simulink model "F16ASYM_Controlled_ACC"  (R2012b)
settings: Solver=ode3  SolverMode=SingleTasking  StartTime=0.0  StopTime=inf  FixedStep=T_sim  RelTol=1e-3
InitFcn:
  | load('NN_c_weights_Last_stable.mat')
values from neighbouring files (symbols this model uses):
  a1 = fitresult.p1    [Stall_protection.m]
  alpha_map_eval = ones(size(M_eval))*NaN    [Auto_trim_aid.m]    (also in Autotrim_maps.mat = [nan nan 0.277598136245 0.119432432992 0.0579479097061 0.027)
  beta_map_eval = ones(size(M_eval))*NaN    [Auto_trim_aid.m]    (also in Autotrim_maps.mat = [nan nan -0.00151549403324 0.00117807579006 -0.0052086799721)
  C_L_0 = fitresult.p2    [Stall_protection.m]
  G_eval = NaN*ones(size(M_sq,2),size(H_sq,2))    [Stall_protection.m]
  H_sq = unique(sort(H_sq))    [Stall_protection.m]
  H_sq_autotrim = min( F_envelope.H_1g):2000:max(F_envelope.H_1g)    [Auto_trim_aid.m]    (also in Autotrim_maps.mat = [0 2000 4000 6000 8000 10000 12000 14000 16000 18000])
  K_b_ACC = params(3)    [Cost_function.m]
  K_b_q = params(4)    [Cost_function.m]
  learning = 20    [Scheduling_desing.m]
  M_sq = unique(sort(M_sq))    [Stall_protection.m]
  M_sq_autotrim = 0:0.1:max(F_envelope.M_1g)    [Auto_trim_aid.m]    (also in Autotrim_maps.mat = [0 0.1 0.2 0.3 0.4 0.5 0.6 0.7 0.8 0.9 1 1.1 ... (21 element)
  Model_used_flag = 1    [Scheduling_desing.m]
  reg_param = 1    [Scheduling_desing.m]
  T_sim = 0.04    [Run_me.m]    (also in Scheduling_desing.m = 0.02)
  tau_ACC = params(1)    [Cost_function.m]
  tau_q = params(2)    [Cost_function.m]
  V_Comp_A_w_z_last = [-0.043311742939 0.0085685727899 -0.0213735657625 0.0330213821126 -0.0306555996667 -0.00573122365227 -0.0106441480787 0.0329440631876 0.0177121952361 -0.0290685435098 -0.0181457235686 -0.0361990502411 ... (1250 elements, 50x25)]    [NN_c_weights_Last_stable.mat]
  V_Comp_last = [-0.0421958473648 0.0184516098779 -0.0436695953504 -0.041154016657 0.00216882652165 -0.0388561228631 0.0327521861474 0.0326079628857 0.0227071838361 -0.0338588476214 0.0161615063846 0.00186003522421 ... (1250 elements, 50x25)]    [NN_c_weights_Last_stable.mat]
  velocity = M_eval(I,J)*a    [Auto_trim_aid.m]    (also in Scheduling_desing.m = M_eval_sche(I,J)*a)
  W_Comp_A_w_z_last = [-0.00689921461652 0.00234704735165 -0.000126421245896 0.00121944724496 6.17702028018e-05 -0.000422762754226 -0.000228913732743 -1.1618795843e-05 7.94007436465e-05 0.000588815786054 2.98617078429e-05 -0.00020420127191 ... (153 elements, 3x51)]    [NN_c_weights_Last_stable.mat]
  W_Comp_last = [-0.00864477030284 0.000183920433695 -0.000300268209456 0.00178165628538 -0.000144806488148 -0.000715209966 -0.000733452792184 5.9552378004e-05 0.000293789747621 0.00184648331608 -0.000150090451416 -0.000741280397229 ... (153 elements, 3x51)]    [NN_c_weights_Last_stable.mat]
undefined symbols (not defined in the file or in its folder): B, DiscIntNeverNeededParam, fi_flag_Simulink, k_B, m_B, sigbuilder_block, Stall_curve, Theta_1_roll_last, Theta_2_roll_last, Theta_3_roll_last, trim_control, trim_state, trim_throttle, V_long_lastA_w_z, V_long_lastAoA, V_roll_last, V_roll_lastMOD, V_yaw_last, W_long_lastA_w_z, W_long_lastAoA, W_roll_last, W_roll_lastMOD, W_yaw_last
libraries: Adaptive_FaultTolerantControl x43, F16_Actuator_Library x14, dspsigops x13, simulink x8, dsparch4 x6, simulink_extras x5, aerolibatmos2 x5, aerolibtransform2 x5, dspmtrx3 x3, qcatlib x2, dspvision x2, dspsnks4 x2
(part 9 of 10)

== system F16ASYM_Controlled_ACC/Primary Controller/P controller + adaptive Crossed NN/Longitudinal Controller: AoA or A_w_z/Longitudinal controller in A_w_z/Accel rate --> AoA rate! ==
  All_meas : Inport
  1/a_1 : Gain  Gain=1/a1
  Bus Selector : BusSelector  OutputSignals=signal2.q (Pa)
  Divide : Product  Inputs=**
  Divide2 : Product  Inputs=*/
  S : Constant  Value=27.87
  mass : Constant  Value=9295.44
  A_w  to AoA rates factor : Outport
  wires:
  1/a_1/1 -> A_w  to AoA rates factor/1
  All_meas/1 -> Bus Selector/1
  Divide2/1 -> 1/a_1/1
  Divide/1 -> Divide2/2
  mass/1 -> Divide2/1
  Bus Selector/1 -> Divide/2  "<q (Pa)>"
  S/1 -> Divide/1

== system F16ASYM_Controlled_ACC/Primary Controller/P controller + adaptive Crossed NN + AWU+Lim /Longitudinal Controller: AoA or A_w_z/Longitudinal controller in A_w_z/Accel rate --> AoA rate! ==
  All_meas : Inport
  1/a_1 : Gain  Gain=1/a1
  Bus Selector : BusSelector  OutputSignals=signal2.q (Pa)
  Divide : Product  Inputs=**
  Divide2 : Product  Inputs=*/
  S : Constant  Value=27.87
  mass : Constant  Value=9295.44
  A_w  to AoA rates factor : Outport
  wires:
  S/1 -> Divide/1
  Bus Selector/1 -> Divide/2  "<q (Pa)>"
  mass/1 -> Divide2/1
  Divide/1 -> Divide2/2
  Divide2/1 -> 1/a_1/1
  All_meas/1 -> Bus Selector/1
  1/a_1/1 -> A_w  to AoA rates factor/1

== matlab function F16ASYM_Controlled_ACC/P controller + adaptive Crossed NN + AWU+Lim    in ACC /Complete crossed On-line (adaptive) multi-layer NN: A_w_z/Cross NN A_w_z ==
  data: X_bar input size=[25,1]; v_ad_comp output; e input; Factor_F input; K_roll input; Ks_long input; Ks_yaw input; B input; Learnign_rate input size=1; Reg_param input size=1; AWU input; W input size=[3,51]; V input size=[50,25]; v_ad output; Z_norm_unit output; T_sim parameter; W_update output; V_update output
function [v_ad_comp,v_ad,Z_norm_unit,W_update,V_update]  = Cross_NN(X_bar,e,Factor_F, K_roll,Ks_long,Ks_yaw,B,Learnign_rate,Reg_param,AWU,W,V,T_sim)

%% Compute prelimiary parametes
% Compute P with regular Lyapunov equation solution
P_roll=1/K_roll;
P_long =  [   1/Ks_long(1) , Factor_F/(Ks_long(1)^2+Ks_long(1)*Ks_long(2));
     1/(Ks_long(1)^2+Ks_long(1)*Ks_long(2)) ,(Ks_long(1)^2+Ks_long(1)*Ks_long(2)+Factor_F^2)/(Ks_long(2)^2*Ks_long(1)+Ks_long(2)*Ks_long(1)^2) ];
P_yaw = [   1/Ks_yaw(1) , 1/(Ks_yaw(1)^2+Ks_yaw(1)*Ks_yaw(2));
     1/(Ks_yaw(1)^2+Ks_yaw(1)*Ks_yaw(2)) ,(Ks_yaw(1)^2+Ks_yaw(1)*Ks_yaw(2)+1)/(Ks_yaw(2)^2*Ks_yaw(1)+Ks_yaw(2)*Ks_yaw(1)^2) ];
 
P = blkdiag(P_roll,P_long,P_yaw);

% % % % Compute P with on-line Lyapunov equation solution
% % % CROSS = 0;
% % % A = [ -K_roll,0,CROSS,0,0;0,-Ks_long(1),1,0,0;
% % %     0,0,-Ks_long(2),0,0;0,0,0,-Ks_yaw(1),Factor_F;0,0,0,0,-Ks_yaw(2)];
% % % 
% % % coder.extrinsic('lyap')
% % % P = A;
% % % P = lyap(A,2*diag(ones(5,1)));



K_awu = 1.2;
zeta= e'*P*B;


% Introduce Anti-windup
zeta = zeta - K_awu*AWU'.*T_sim; 

% Convergence limitation
if norm(zeta)>2/(T_sim*Learnign_rate*Reg_param)
    zeta = (zeta./norm(zeta)).*(1.8/(T_sim*Learnign_rate*Reg_param));
end

%% Feedforward
z = V*X_bar;
s=sigmoid(V*X_bar);

sigma = [1 ; s ];
% v_ad = W*sigma;

sigma_grad = (sigma.*(ones(size(sigma))-sigma));

%% Compute the gradients or adaptation laws
Gamma_w= Learnign_rate; % W learnign rate
Gamma_v= Learnign_rate; %V learning rate
lambda = Reg_param;

V_dot=zeros(size(V));
W_dot=zeros(size(W));

W_dot= -Gamma_w*(  (sigma - sigma_grad.*[1;z] )*zeta  )';
W_dot(:,2:end)= W_dot(:,2:end) - Gamma_w*lambda*norm(zeta)*(W(:,2:end));

M = W'*zeta'.*sigma_grad ;
V_dot= -Gamma_v*( M(2:end)*X_bar'  );
V_dot(:,2:end)= V_dot(:,2:end) - Gamma_v*lambda*norm(zeta).*V(:,2:end);

% % % Other way: Based on notes of Andrew NG
% % 
% % delta2=W'*zeta'.*sigma_grad;
% % 
% % V_dot = - Gamma_v*( delta2(2:end)*X_bar');
% % V_dot(:,2:end)= V_dot(:,2:end) - Gamma_v*lambda*norm(zeta).*V(:,2:end);
% % 
% % W_dot = - Gamma_w*( sigma*zeta)';
% % W_dot(:,2:end)= W_dot(:,2:end) - Gamma_w*lambda*norm(zeta)*(W(:,2:end));



%% Adaptation
W_update = W + T_sim*W_dot;
V_update = V + T_sim*V_dot;
% 
%% Re-compute v_ad

s=sigmoid(V_update*X_bar);

sigma = [1 ; s(:,1) ];
v_ad = W_update*sigma;

%% Compute v_ad_comp
Z = [ V,zeros(size(V,1),size(W,2));
    zeros(size(W,1),size(V,2)),W];
    
Z_norm = norm(Z,'fro');
Z_max = 2*min(size(W,1),size(W,2) )*min( size(V,1),size(V,2) );
Z_norm_unit = Z_norm;

K_r0= 0;
K_r1= 0;
v_r0 = -K_r0*zeta';
v_r1 = -K_r1*(Z_norm+Z_max)*zeta';

v_ad_comp = v_ad + v_r1 +v_r0;

% % % Normalization of matrices
% % if Z_norm>Z_max
% %     V = (V.*Z_max)./Z_norm;
% %     W = (W.*Z_max)./Z_norm;
% % end
end

== matlab function F16ASYM_Controlled_ACC/Primary Controller/P  + Crossed NN + AWU+Lim + hand-over/P controller + adaptive Crossed NN + AWU+Lim   in AoA/Physical limitation/max deflections estimator ==
  data: v_comm input; max_defl output; B parameter
function max_defl = Max_defl(v_comm,B)
sup_limit = [24,24,21,21,29,25,25];
inf_limit = [-24,-24,-21,-21,-29,0,0];

def=B;
for i=1:3
    def(i,:) = B(i,:).*sign(v_comm(i));
end
def_avg = mean(def,1);

max_defl = zeros(7,1);
for i=1:7
    if def_avg(1,i)>0
        max_defl(i) = sup_limit(i);
    else
        max_defl(i) = inf_limit(i);
    end
end

== matlab function F16ASYM_Controlled_ACC/Primary Controller/P  + Crossed NN + AWU+Lim + hand-over/P controller + adaptive Crossed NN + AWU+Lim    in ACC /Physical limitation/max deflections estimator ==
  data: v_comm input; max_defl output; B parameter
function max_defl = Max_defl(v_comm,B)
sup_limit = [24,24,21,21,29,25,25];
inf_limit = [-24,-24,-21,-21,-29,0,0];

def=B;
for i=1:3
    def(i,:) = B(i,:).*sign(v_comm(i));
end
def_avg = mean(def,1);

max_defl = zeros(7,1);
for i=1:7
    if def_avg(1,i)>0
        max_defl(i) = sup_limit(i);
    else
        max_defl(i) = inf_limit(i);
    end
end

== matlab function F16ASYM_Controlled_ACC/P controller + adaptive Crossed NN + AWU+Lim    in ACC /Sigmoid /MATLAB Function ==
  data: u input; y output; a input
function y = sigmoid_a(u,a)

y = 2.0 ./ (1.0 + exp(-a*u(1:3)))-1;

== system F16ASYM_Controlled_ACC/Primary Controller/P controller + adaptive Crossed NN + AWU+Lim /Longitudinal Controller: AoA or A_w_z/Longitudinal controller in A_w_z/Stall protection ==
  alpha_dot des : Inport
  All meas : Inport  Port=2
  Bus Selector : BusSelector  OutputSignals=signal1.AoA meas (rad)
  MATLAB Function : MATLAB Function  TreatAsAtomicUnit=on
  AoA des : Outport
  wires:
  alpha_dot des/1 -> MATLAB Function/1(alpha_dot)
  MATLAB Function/1(alpha_dot_out) -> AoA des/1
  All meas/1 -> Bus Selector/1
  Bus Selector/1 -> MATLAB Function/2(alpha)  "<AoA meas (rad)>"

== system F16ASYM_Controlled_ACC/Primary Controller/P controller + adaptive Isolated NN/Longitudinal Controller: AoA or A_w_z/Longitudinal controller in A_w_z/Accel rate --> AoA rate! ==
  All_meas : Inport
  1/a_1 : Gain  Gain=1/a1
  Bus Selector : BusSelector  OutputSignals=signal2.q (Pa)
  Divide : Product  Inputs=**
  Divide2 : Product  Inputs=*/
  S : Constant  Value=27.87
  mass : Constant  Value=9295.44
  A_w  to AoA rates factor : Outport
  wires:
  S/1 -> Divide/1
  Bus Selector/1 -> Divide/2  "<q (Pa)>"
  mass/1 -> Divide2/1
  Divide/1 -> Divide2/2
  Divide2/1 -> 1/a_1/1
  All_meas/1 -> Bus Selector/1
  1/a_1/1 -> A_w  to AoA rates factor/1

== system F16ASYM_Controlled_ACC/Primary Controller/P controller + adaptive Isolated NN/On-line (adaptive) multi-layer NNs/Long Chanel/Long HL NN A_w_z ==
  note: Be careful with dimensions of inputs!!!
      | NORMALIZATION!!!
  v_ad^ prev : Inport
  Long_chanel vars : Inport  Port=2
  All_meas : Inport  Port=3
  Long_learning rate : Inport  Port=4
  Long reg param : Inport  Port=5
  Bus Selector1 : BusSelector  OutputSignals=A_chanel vars.A_err,q_chanel_vars.q_err,A_chanel vars.A_sf,A_chanel vars.A_sf_dot,q_chanel_vars.q_sf_dot,A_chanel vars.K_b_A,q_chanel_vars.K_b_q,A_chanel vars.FactorF
  Bus Selector2 : BusSelector  OutputSignals=signal1.Alt meas (m),signal2.Mach
  Constant : Constant
  Constant1 : Constant  Value=[0;1]
  Divide : Product  Inputs=**
  Long NN : MATLAB Function  TreatAsAtomicUnit=on
  Memory2 : Memory  X0=V_long_lastA_w_z
  Memory3 : Memory  X0=W_long_lastA_w_z
  Mux : Mux  Inputs=10
  Mux1 : Mux  Inputs=2
  Mux2 : Mux  Inputs=2
  Scope : Scope
      settings: YMin=0  YMax=0.003  SaveName=ScopeData13
  Terminator : Terminator
  Terminator1 : Terminator
  To Workspace : ToWorkspace  VariableName=V_long_lastA_w_z  SampleTime=-1
      settings: MaxDataPoints=1
  To Workspace1 : ToWorkspace  VariableName=W_long_lastA_w_z  SampleTime=-1
      settings: MaxDataPoints=1
  dim-less : Gain  Gain=T_sim
  dim-less1 : Gain  Gain=T_sim^2
  scaling : Gain  Gain=1/15000
  scaling1 : Gain  Gain=1/(9*9.81)
  scaling2 : Gain  Gain=1/(9*9.81)
  scaling3 : Gain  Gain=1/(9*9.81)
  v_ad_comp : Outport
  wires:
  Long NN/2(v_ad) -> Terminator/1
  Long NN/5(V_update) -> To Workspace/1, Memory2/1
  v_ad^ prev/1 -> Mux/10
  [Ks] -> Long NN/4(Ks)
  Constant1/1 -> Long NN/5(B)
  Memory3/1 -> Long NN/8(W)
  Memory2/1 -> Long NN/9(V)
  Long NN/4(W_update) -> To Workspace1/1, Memory3/1
  Long NN/1(v_ad_comp) -> v_ad_comp/1
  Mux/1 -> Scope/1, Long NN/1(X_bar)
  Long_chanel vars/1 -> Bus Selector1/1
  Long_learning rate/1 -> Long NN/6(Long_learnign_rate)
  Long reg param/1 -> Long NN/7(Long_reg_param)
  Constant/1 -> Mux/1
  All_meas/1 -> Bus Selector2/1
  Bus Selector2/1 -> scaling/1  "<Alt meas (m)>"
  Divide/1 -> Mux/4
  scaling/1 -> Mux/2
  Bus Selector2/2 -> Mux/3, Divide/2, Divide/1  "<Mach>"
  Bus Selector1/1 -> Mux1/1, scaling2/1  "<A_err>"
  Bus Selector1/2 -> Mux1/2, Mux/6  "<q_err>"
  Bus Selector1/3 -> scaling1/1  "<A_sf>"
  Bus Selector1/4 -> dim-less/1  "<A_sf_dot>"
  Bus Selector1/5 -> dim-less1/1  "<q_sf_dot>"
  Mux1/1 -> Long NN/2(e)  "e"
  Bus Selector1/7 -> Mux2/2  "<K_b_q>"
  Bus Selector1/6 -> Mux2/1  "<K_b_A>"
  Mux2/1 -> [Ks]
  Bus Selector1/8 -> Long NN/3(F)  "<FactorF>"
  scaling2/1 -> Mux/5
  scaling1/1 -> Mux/7
  scaling3/1 -> Mux/8
  Long NN/3(Z_norm_unit) -> Terminator1/1
  dim-less/1 -> scaling3/1
  dim-less1/1 -> Mux/9

== system F16ASYM_Controlled_ACC/Primary Controller/P controller + adaptive Isolated NN/On-line (adaptive) multi-layer NNs/Long Chanel/Long HL NN AoA ==
  note: Be careful with dimensions of inputs!!!
      | NORMALIZATION!!!
  v_ad^ prev : Inport
  Long_chanel vars : Inport  Port=2
  All_meas : Inport  Port=3
  Long_learning rate : Inport  Port=4
  Long reg param : Inport  Port=5
  Bus Selector1 : BusSelector  OutputSignals=alpha_chanel vars.alpha_err,q_chanel_vars.q_err,alpha_chanel vars.alpha_sf,alpha_chanel vars.alpha_sf_dot,q_chanel_vars.q_sf_dot,alpha_chanel vars.K_b_alpha,q_chanel_vars.K_b_q
  Bus Selector2 : BusSelector  OutputSignals=signal1.Alt meas (m),signal2.Mach
  Constant : Constant
  Constant1 : Constant  Value=[0;1]
  Display : Display
  Divide : Product  Inputs=**
  Gain : Gain  Gain=1/15000
  Long NN : MATLAB Function  TreatAsAtomicUnit=on
  Memory2 : Memory  X0=V_long_lastAoA
  Memory3 : Memory  X0=W_long_lastAoA
  Mux : Mux  Inputs=10
  Mux1 : Mux  Inputs=2
  Mux2 : Mux  Inputs=2
  Scope : Scope
      settings: YMin=-0.7  YMax=1  SaveName=ScopeData18
  Terminator : Terminator
  Terminator1 : Terminator
  To Workspace : ToWorkspace  VariableName=V_long_lastAoA  SampleTime=-1
      settings: MaxDataPoints=1
  To Workspace1 : ToWorkspace  VariableName=W_long_lastAoA  SampleTime=-1
      settings: MaxDataPoints=1
  dem-less : Gain  Gain=T_sim
  dem-less1 : Gain  Gain=T_sim^2
  v_ad_comp : Outport
  wires:
  Long NN/2(v_ad) -> Terminator/1
  Long NN/5(V_update) -> To Workspace/1, Memory2/1
  v_ad^ prev/1 -> Mux/10
  [Ks] -> Long NN/3(Ks)
  Constant1/1 -> Long NN/4(B)
  Memory3/1 -> Long NN/7(W)
  Memory2/1 -> Long NN/8(V)
  Long NN/4(W_update) -> To Workspace1/1, Memory3/1
  Long NN/1(v_ad_comp) -> v_ad_comp/1
  Long_chanel vars/1 -> Bus Selector1/1
  Long_learning rate/1 -> Long NN/5(Long_learnign_rate)
  Long reg param/1 -> Long NN/6(Long_reg_param)
  Constant/1 -> Mux/1
  All_meas/1 -> Bus Selector2/1
  Bus Selector2/1 -> Gain/1  "<Alt meas (m)>"
  Divide/1 -> Mux/4
  Gain/1 -> Mux/2
  Bus Selector2/2 -> Mux/3, Divide/2, Divide/1  "<Mach>"
  Bus Selector1/1 -> Mux1/1, Mux/5  "<alpha_err>"
  Bus Selector1/2 -> Mux1/2, Mux/6  "<q_err>"
  Bus Selector1/3 -> Mux/7  "<alpha_sf>"
  Bus Selector1/4 -> dem-less/1  "<alpha_sf_dot>"
  Bus Selector1/5 -> dem-less1/1  "<q_sf_dot>"
  Mux1/1 -> Long NN/2(e)  "e"
  Bus Selector1/7 -> Mux2/2  "<K_b_q>"
  Bus Selector1/6 -> Mux2/1  "<K_b_alpha>"
  Mux2/1 -> [Ks]
  Long NN/3(Z_norm_unit) -> Terminator1/1
  Mux/1 -> Scope/1, Display/1, Long NN/1(X_bar)
  dem-less/1 -> Mux/8
  dem-less1/1 -> Mux/9

== system F16ASYM_Controlled_ACC/Primary Controller/P controller + adaptive Isolated NN/On-line (adaptive) multi-layer NNs/Roll NN/Roll 1HL NN ==
  note: Be careful with dimensions of inputs!!!
      | NORMALIZATION!!!
  v_ad^ prev : Inport
  p_chanel vars : Inport  Port=2
  All_meas : Inport  Port=3
  Roll_learning rate : Inport  Port=4
  Roll reg param : Inport  Port=5
  Bus Selector1 : BusSelector  OutputSignals=p_err,p_sf,p_sf_dot,K_b_p
  Bus Selector2 : BusSelector  OutputSignals=signal1.Alt meas (m),signal2.Mach,signal1.AoA meas (rad),signal1.SS meas (rad),signal1.omega_b meas (rad/s)
  Constant : Constant
  Constant1 : Constant
  Constant2 : Constant
  Display : Display
  Divide : Product  Inputs=**
  Divide1 : Product  Inputs=**
  Divide2 : Product  Inputs=*/
  Memory2 : Memory  X0=V_roll_last
  Memory3 : Memory  X0=W_roll_last
  Mux : Mux  Inputs=12
  Roll NN : MATLAB Function  TreatAsAtomicUnit=on
  Scope : Scope
      settings: YMin=-0.5  YMax=6  SaveName=ScopeData15
  Selector : Selector  InputPortWidth=3  IndexOptions=Index vector (dialog)  Indices=3  OutputSizes=1
  Terminator : Terminator
  Terminator1 : Terminator
  To Workspace : ToWorkspace  VariableName=V_roll_last  SampleTime=-1
      settings: MaxDataPoints=1
  To Workspace1 : ToWorkspace  VariableName=W_roll_last  SampleTime=-1
      settings: MaxDataPoints=1
  dem-less : Gain  Gain=T_sim
  dim-less : Gain  Gain=1/15000
  v_ad_comp : Outport
  wires:
  Constant2/1 -> Divide2/1
  Bus Selector1/4 -> Divide2/2  "<K_b_p>"
  Divide2/1 -> [P]
  Roll NN/2(v_ad) -> Terminator/1
  Roll NN/5(V_update) -> To Workspace/1, Memory2/1
  v_ad^ prev/1 -> Mux/12
  [P] -> Roll NN/3(P)
  Constant1/1 -> Roll NN/4(B)
  Memory3/1 -> Roll NN/7(W)
  Memory2/1 -> Roll NN/8(V)
  Roll NN/4(W_update) -> To Workspace1/1, Memory3/1
  Roll NN/1(v_ad_comp) -> v_ad_comp/1
  Mux/1 -> Roll NN/1(X_bar), Scope/1, Display/1
  Bus Selector1/1 -> Mux/9, Roll NN/2(e)  "<p_err>"
  Bus Selector1/3 -> dem-less/1  "<p_sf_dot>"
  Bus Selector1/2 -> Mux/10  "<p_sf>"
  p_chanel vars/1 -> Bus Selector1/1
  Roll_learning rate/1 -> Roll NN/5(Roll_learnign_rate)
  Roll reg param/1 -> Roll NN/6(Roll_reg_param)
  Constant/1 -> Mux/1
  All_meas/1 -> Bus Selector2/1
  Bus Selector2/1 -> dim-less/1  "<Alt meas (m)>"
  Divide/1 -> Mux/4
  Bus Selector2/3 -> Divide1/2, Divide1/1, Mux/5  "<AoA meas (rad)>"
  Divide1/1 -> Mux/6
  Bus Selector2/4 -> Mux/7  "<SS meas (rad)>"
  dim-less/1 -> Mux/2
  Bus Selector2/5 -> Selector/1  "<omega_b meas (rad/s)>"
  Selector/1 -> Mux/8
  Bus Selector2/2 -> Divide/2, Divide/1, Mux/3  "<Mach>"
  Roll NN/3(Z_norm_unit) -> Terminator1/1
  dem-less/1 -> Mux/11

== system F16ASYM_Controlled_ACC/Primary Controller/P controller + adaptive Isolated NN/On-line (adaptive) multi-layer NNs/Roll NN/Roll 2HL NN ==
  note: Be careful with dimensions of inputs!!!
      | NORMALIZATION!!!
  v_ad^ prev : Inport
  p_chanel vars : Inport  Port=2
  All_meas : Inport  Port=3
  Roll_learning rate : Inport  Port=4
  Roll reg param : Inport  Port=5
  " " : ToWorkspace  VariableName=Theta_3_roll_last  SampleTime=-1
      settings: MaxDataPoints=1
  "  " : Memory  X0=Theta_3_roll_last
  "   " : Memory  X0=Theta_2_roll_last
  B : Constant
  Bus Selector1 : BusSelector  OutputSignals=p_err,p_sf,p_sf_dot,K_b_p
  Bus Selector2 : BusSelector  OutputSignals=signal1.Alt meas (m),signal2.Mach,signal1.AoA meas (rad),signal1.SS meas (rad),signal1.omega_b meas (rad/s)
  Constant : Constant
  Constant2 : Constant
  Display : Display
  Divide : Product  Inputs=**
  Divide1 : Product  Inputs=**
  Divide2 : Product  Inputs=*/
  Gain : Gain  Gain=1/15000
  Memory2 : Memory  X0=Theta_1_roll_last
  Mux : Mux  Inputs=12
  Roll Multilayer NN : MATLAB Function  TreatAsAtomicUnit=on
  Scope : Scope
      settings: YMin=-14  YMax=4  SaveName=ScopeData16
  Selector : Selector  InputPortWidth=3  IndexOptions=Index vector (dialog)  Indices=3  OutputSizes=1
  Terminator : Terminator
  Terminator1 : Terminator
  To Workspace : ToWorkspace  VariableName=Theta_1_roll_last  SampleTime=-1
      settings: MaxDataPoints=1
  To Workspace1 : ToWorkspace  VariableName=Theta_2_roll_last  SampleTime=-1
      settings: MaxDataPoints=1
  dem-less : Gain  Gain=T_sim
  v_ad_comp : Outport
  wires:
  p_chanel vars/1 -> Bus Selector1/1
  Bus Selector1/2 -> Mux/10  "<p_sf>"
  Bus Selector1/3 -> dem-less/1  "<p_sf_dot>"
  Bus Selector1/1 -> Mux/9, Roll Multilayer NN/2(e)  "<p_err>"
  Constant/1 -> Mux/1
  All_meas/1 -> Bus Selector2/1
  Bus Selector2/1 -> Gain/1  "<Alt meas (m)>"
  Divide/1 -> Mux/4
  Bus Selector2/3 -> Divide1/2, Divide1/1, Mux/5  "<AoA meas (rad)>"
  Divide1/1 -> Mux/6
  Bus Selector2/4 -> Mux/7  "<SS meas (rad)>"
  Gain/1 -> Mux/2
  Bus Selector2/5 -> Selector/1  "<omega_b meas (rad/s)>"
  Selector/1 -> Mux/8
  Roll Multilayer NN/1(v_ad_comp) -> v_ad_comp/1
  "   "/1 -> Roll Multilayer NN/8(Theta_2)
  B/1 -> Roll Multilayer NN/4(B)
  [P] -> Roll Multilayer NN/3(P)
  v_ad^ prev/1 -> Mux/12
  Roll Multilayer NN/4(Theta_1_update) -> To Workspace/1, Memory2/1
  Roll Multilayer NN/2(v_ad) -> Terminator/1
  Divide2/1 -> [P]
  Bus Selector1/4 -> Divide2/2  "<K_b_p>"
  Constant2/1 -> Divide2/1
  Bus Selector2/2 -> Divide/2, Divide/1, Mux/3  "<Mach>"
  Roll Multilayer NN/6(Theta_3_update) -> "  "/1, " "/1
  "  "/1 -> Roll Multilayer NN/9(Theta_3)
  Roll Multilayer NN/5(Theta_2_update) -> To Workspace1/1, "   "/1
  Memory2/1 -> Roll Multilayer NN/7(Theta_1)
  Roll_learning rate/1 -> Roll Multilayer NN/5(Roll_learnign_rate)
  Roll reg param/1 -> Roll Multilayer NN/6(Roll_reg_param)
  Mux/1 -> Display/1, Scope/1, Roll Multilayer NN/1(X_bar)
  Roll Multilayer NN/3(Z_norm_unit) -> Terminator1/1
  dem-less/1 -> Mux/11

== system F16ASYM_Controlled_ACC/Primary Controller/P controller + adaptive Isolated NN/On-line (adaptive) multi-layer NNs/Yaw Chanel/Yaw HL NN ==
  note: Be careful with dimensions of inputs!!!
      | NORMALIZATION!!!
  v_ad^ prev : Inport
  Yaw_chanel vars : Inport  Port=2
  All_meas : Inport  Port=3
  Yaw_learning rate : Inport  Port=4
  Yaw reg param : Inport  Port=5
  Bus Selector1 : BusSelector  OutputSignals=beta_chanel vars.beta_err,r_chanel vars.r_err,beta_chanel vars.beta_sf,beta_chanel vars.beta_sf_dot,r_chanel vars.r_sf_dot,beta_chanel vars.K_b_beta,r_chanel vars.K_b_r
  Bus Selector2 : BusSelector  OutputSignals=signal1.Alt meas (m),signal2.Mach,signal1.AoA meas (rad),signal1.Euler meas (rad)
  Constant : Constant
  Constant1 : Constant  Value=[0;1]
  Display : Display
  Divide : Product  Inputs=**
  Gain : Gain  Gain=1/15000
  Memory2 : Memory  X0=V_yaw_last
  Memory3 : Memory  X0=W_yaw_last
  Mux : Mux  Inputs=12
  Mux1 : Mux  Inputs=2
  Mux2 : Mux  Inputs=2
  Scope : Scope
      settings: YMin=-0.25  YMax=3.75  SaveName=ScopeData17
  Selector : Selector  InputPortWidth=3  IndexOptions=Index vector (dialog)  Indices=1  OutputSizes=1
  Terminator : Terminator
  Terminator1 : Terminator
  To Workspace : ToWorkspace  VariableName=V_yaw_last  SampleTime=-1
      settings: MaxDataPoints=1
  To Workspace1 : ToWorkspace  VariableName=W_yaw_last  SampleTime=-1
      settings: MaxDataPoints=1
  Yaw NN : MATLAB Function  TreatAsAtomicUnit=on
  dem-less1 : Gain  Gain=T_sim
  dem-less2 : Gain  Gain=T_sim^2
  v_ad_comp : Outport
  wires:
  Mux2/1 -> [Ks]
  Bus Selector1/6 -> Mux2/1  "<K_b_beta>"
  Bus Selector1/7 -> Mux2/2  "<K_b_r>"
  Mux1/1 -> Yaw NN/2(e)  "e"
  Divide/1 -> Mux/4
  Bus Selector2/1 -> Gain/1  "<Alt meas (m)>"
  All_meas/1 -> Bus Selector2/1
  Constant/1 -> Mux/1
  Yaw reg param/1 -> Yaw NN/6(Long_reg_param)
  Yaw_learning rate/1 -> Yaw NN/5(Long_learnign_rate)
  Yaw_chanel vars/1 -> Bus Selector1/1
  Yaw NN/1(v_ad_comp) -> v_ad_comp/1
  Yaw NN/4(W_update) -> Memory3/1, To Workspace1/1
  Memory2/1 -> Yaw NN/8(V)
  Memory3/1 -> Yaw NN/7(W)
  Constant1/1 -> Yaw NN/4(B)
  [Ks] -> Yaw NN/3(Ks)
  v_ad^ prev/1 -> Mux/12
  Yaw NN/5(V_update) -> Memory2/1, To Workspace/1
  Yaw NN/2(v_ad) -> Terminator/1
  Bus Selector2/4 -> Selector/1  "<Euler meas (rad)>"
  Gain/1 -> Mux/2
  Bus Selector2/2 -> Divide/2, Divide/1, Mux/3  "<Mach>"
  Bus Selector2/3 -> Mux/5  "<AoA meas (rad)>"
  Selector/1 -> Mux/6
  Bus Selector1/5 -> dem-less2/1  "<r_sf_dot>"
  Bus Selector1/2 -> Mux1/2, Mux/8  "<r_err>"
  Bus Selector1/4 -> dem-less1/1  "<beta_sf_dot>"
  Bus Selector1/1 -> Mux1/1, Mux/7  "<beta_err>"
  Bus Selector1/3 -> Mux/9  "<beta_sf>"
  Mux/1 -> Display/1, Scope/1, Yaw NN/1(X_bar)
  Yaw NN/3(Z_norm_unit) -> Terminator1/1
  dem-less1/1 -> Mux/10
  dem-less2/1 -> Mux/11

== system F16ASYM_Controlled_ACC/Primary Controller/P controller + adaptive Isolated NN/On-line (adaptive) multi-layer NNs SIMPL/Long Chanel/Long HL NN A_w_z ==
  note: Be careful with dimensions of inputs!!!
      | NORMALIZATION!!!
  v_ad^ prev : Inport
  Long_chanel vars : Inport  Port=2
  All_meas : Inport  Port=3
  Long_learning rate : Inport  Port=4
  Long reg param : Inport  Port=5
  Bus Selector1 : BusSelector  OutputSignals=A_chanel vars.A_err,q_chanel_vars.q_err,A_chanel vars.A_sf,A_chanel vars.A_sf_dot,q_chanel_vars.q_sf_dot,A_chanel vars.K_b_A,q_chanel_vars.K_b_q,A_chanel vars.FactorF
  Bus Selector2 : BusSelector  OutputSignals=signal1.Alt meas (m),signal2.Mach
  Constant : Constant
  Constant1 : Constant  Value=[0;1]
  Divide : Product  Inputs=**
  Long NN : MATLAB Function  TreatAsAtomicUnit=on
  Memory2 : Memory  X0=V_long_lastA_w_z
  Memory3 : Memory  X0=W_long_lastA_w_z
  Mux : Mux  Inputs=10
  Mux1 : Mux  Inputs=2
  Mux2 : Mux  Inputs=2
  Scope : Scope
      settings: YMin=0  YMax=0.003  SaveName=ScopeData13
  Terminator : Terminator
  Terminator1 : Terminator
  To Workspace : ToWorkspace  VariableName=V_long_lastA_w_z  SampleTime=-1
      settings: MaxDataPoints=1
  To Workspace1 : ToWorkspace  VariableName=W_long_lastA_w_z  SampleTime=-1
      settings: MaxDataPoints=1
  dim-less : Gain  Gain=T_sim
  dim-less1 : Gain  Gain=T_sim^2
  scaling : Gain  Gain=1/15000
  scaling1 : Gain  Gain=1/(9*9.81)
  scaling2 : Gain  Gain=1/(9*9.81)
  scaling3 : Gain  Gain=1/(9*9.81)
  v_ad_comp : Outport
  wires:
  dim-less1/1 -> Mux/9
  dim-less/1 -> scaling3/1
  Long NN/3(Z_norm_unit) -> Terminator1/1
  scaling3/1 -> Mux/8
  scaling1/1 -> Mux/7
  scaling2/1 -> Mux/5
  Bus Selector1/8 -> Long NN/3(F)  "<FactorF>"
  Mux2/1 -> [Ks]
  Bus Selector1/6 -> Mux2/1  "<K_b_A>"
  Bus Selector1/7 -> Mux2/2  "<K_b_q>"
  Mux1/1 -> Long NN/2(e)  "e"
  Bus Selector1/5 -> dim-less1/1  "<q_sf_dot>"
  Bus Selector1/4 -> dim-less/1  "<A_sf_dot>"
  Bus Selector1/3 -> scaling1/1  "<A_sf>"
  Bus Selector1/2 -> Mux/6, Mux1/2  "<q_err>"
  Bus Selector1/1 -> scaling2/1, Mux1/1  "<A_err>"
  Bus Selector2/2 -> Divide/1, Divide/2, Mux/3  "<Mach>"
  scaling/1 -> Mux/2
  Divide/1 -> Mux/4
  Bus Selector2/1 -> scaling/1  "<Alt meas (m)>"
  All_meas/1 -> Bus Selector2/1
  Constant/1 -> Mux/1
  Long reg param/1 -> Long NN/7(Long_reg_param)
  Long_learning rate/1 -> Long NN/6(Long_learnign_rate)
  Long_chanel vars/1 -> Bus Selector1/1
  Mux/1 -> Long NN/1(X_bar), Scope/1
  Long NN/1(v_ad_comp) -> v_ad_comp/1
  Long NN/4(W_update) -> Memory3/1, To Workspace1/1
  Memory2/1 -> Long NN/9(V)
  Memory3/1 -> Long NN/8(W)
  Constant1/1 -> Long NN/5(B)
  [Ks] -> Long NN/4(Ks)
  v_ad^ prev/1 -> Mux/10
  Long NN/5(V_update) -> Memory2/1, To Workspace/1
  Long NN/2(v_ad) -> Terminator/1

== system F16ASYM_Controlled_ACC/Primary Controller/P controller + adaptive Isolated NN/On-line (adaptive) multi-layer NNs SIMPL/Long Chanel/Long HL NN AoA ==
  note: Be careful with dimensions of inputs!!!
      | NORMALIZATION!!!
  v_ad^ prev : Inport
  Long_chanel vars : Inport  Port=2
  All_meas : Inport  Port=3
  Long_learning rate : Inport  Port=4
  Long reg param : Inport  Port=5
  Bus Selector1 : BusSelector  OutputSignals=alpha_chanel vars.alpha_err,q_chanel_vars.q_err,alpha_chanel vars.alpha_sf,alpha_chanel vars.alpha_sf_dot,q_chanel_vars.q_sf_dot,alpha_chanel vars.K_b_alpha,q_chanel_vars.K_b_q
  Bus Selector2 : BusSelector  OutputSignals=signal1.Alt meas (m),signal2.Mach
  Constant : Constant
  Constant1 : Constant  Value=[0;1]
  Display : Display
  Divide : Product  Inputs=**
  Gain : Gain  Gain=1/15000
  Long NN : MATLAB Function  TreatAsAtomicUnit=on
  Memory2 : Memory  X0=V_long_lastAoA
  Memory3 : Memory  X0=W_long_lastAoA
  Mux : Mux  Inputs=10
  Mux1 : Mux  Inputs=2
  Mux2 : Mux  Inputs=2
  Scope : Scope
      settings: YMin=-0.7  YMax=1  SaveName=ScopeData18
  Terminator : Terminator
  Terminator1 : Terminator
  To Workspace : ToWorkspace  VariableName=V_long_lastAoA  SampleTime=-1
      settings: MaxDataPoints=1
  To Workspace1 : ToWorkspace  VariableName=W_long_lastAoA  SampleTime=-1
      settings: MaxDataPoints=1
  v_ad_comp : Outport
  wires:
  Mux/1 -> Long NN/1(X_bar), Display/1, Scope/1
  Long NN/3(Z_norm_unit) -> Terminator1/1
  Mux2/1 -> [Ks]
  Bus Selector1/6 -> Mux2/1  "<K_b_alpha>"
  Bus Selector1/7 -> Mux2/2  "<K_b_q>"
  Mux1/1 -> Long NN/2(e)  "e"
  Bus Selector1/5 -> Mux/9  "<q_sf_dot>"
  Bus Selector1/4 -> Mux/8  "<alpha_sf_dot>"
  Bus Selector1/3 -> Mux/7  "<alpha_sf>"
  Bus Selector1/2 -> Mux/6, Mux1/2  "<q_err>"
  Bus Selector1/1 -> Mux/5, Mux1/1  "<alpha_err>"
  Bus Selector2/2 -> Divide/1, Divide/2, Mux/3  "<Mach>"
  Gain/1 -> Mux/2
  Divide/1 -> Mux/4
  Bus Selector2/1 -> Gain/1  "<Alt meas (m)>"
  All_meas/1 -> Bus Selector2/1
  Constant/1 -> Mux/1
  Long reg param/1 -> Long NN/6(Long_reg_param)
  Long_learning rate/1 -> Long NN/5(Long_learnign_rate)
  Long_chanel vars/1 -> Bus Selector1/1
  Long NN/1(v_ad_comp) -> v_ad_comp/1
  Long NN/4(W_update) -> Memory3/1, To Workspace1/1
  Memory2/1 -> Long NN/8(V)
  Memory3/1 -> Long NN/7(W)
  Constant1/1 -> Long NN/4(B)
  [Ks] -> Long NN/3(Ks)
  v_ad^ prev/1 -> Mux/10
  Long NN/5(V_update) -> Memory2/1, To Workspace/1
  Long NN/2(v_ad) -> Terminator/1

== system F16ASYM_Controlled_ACC/Primary Controller/P controller + adaptive Isolated NN/On-line (adaptive) multi-layer NNs SIMPL/Roll NN/Roll 1HL NN ==
  note: Be careful with dimensions of inputs!!!
      | NORMALIZATION!!!
  v_ad^ prev : Inport
  p_chanel vars : Inport  Port=2
  All_meas : Inport  Port=3
  Roll_learning rate : Inport  Port=4
  Roll reg param : Inport  Port=5
  Bus Selector1 : BusSelector  OutputSignals=p_err,p_sf,p_sf_dot,K_b_p
  Bus Selector2 : BusSelector  OutputSignals=signal1.AoA meas (rad),signal1.SS meas (rad),signal1.omega_b meas (rad/s)
  Constant : Constant
  Constant1 : Constant
  Constant2 : Constant
  Display : Display
  Divide2 : Product  Inputs=*/
  Memory2 : Memory  X0=V_roll_lastMOD
  Memory3 : Memory  X0=W_roll_lastMOD
  Mux : Mux  Inputs=8
  Roll NN : MATLAB Function  TreatAsAtomicUnit=on
  Scope : Scope
      settings: YMin=-0.5  YMax=6  SaveName=ScopeData15
  Selector : Selector  InputPortWidth=3  IndexOptions=Index vector (dialog)  Indices=3  OutputSizes=1
  Terminator : Terminator
  Terminator1 : Terminator
  To Workspace : ToWorkspace  VariableName=V_roll_lastMOD  SampleTime=-1
      settings: MaxDataPoints=1
  To Workspace1 : ToWorkspace  VariableName=W_roll_lastMOD  SampleTime=-1
      settings: MaxDataPoints=1
  dem-less : Gain  Gain=T_sim
  v_ad_comp : Outport
  wires:
  dem-less/1 -> Mux/7
  Roll NN/3(Z_norm_unit) -> Terminator1/1
  Selector/1 -> Mux/4
  Bus Selector2/3 -> Selector/1  "<omega_b meas (rad/s)>"
  Bus Selector2/2 -> Mux/3  "<SS meas (rad)>"
  Bus Selector2/1 -> Mux/2  "<AoA meas (rad)>"
  All_meas/1 -> Bus Selector2/1
  Constant/1 -> Mux/1
  Roll reg param/1 -> Roll NN/6(Roll_reg_param)
  Roll_learning rate/1 -> Roll NN/5(Roll_learnign_rate)
  p_chanel vars/1 -> Bus Selector1/1
  Bus Selector1/2 -> Mux/6  "<p_sf>"
  Bus Selector1/3 -> dem-less/1  "<p_sf_dot>"
  Bus Selector1/1 -> Mux/5, Roll NN/2(e)  "<p_err>"
  Mux/1 -> Display/1, Scope/1, Roll NN/1(X_bar)
  Roll NN/1(v_ad_comp) -> v_ad_comp/1
  Roll NN/4(W_update) -> Memory3/1, To Workspace1/1
  Memory2/1 -> Roll NN/8(V)
  Memory3/1 -> Roll NN/7(W)
  Constant1/1 -> Roll NN/4(B)
  [P] -> Roll NN/3(P)
  v_ad^ prev/1 -> Mux/8
  Roll NN/5(V_update) -> Memory2/1, To Workspace/1
  Roll NN/2(v_ad) -> Terminator/1
  Divide2/1 -> [P]
  Bus Selector1/4 -> Divide2/2  "<K_b_p>"
  Constant2/1 -> Divide2/1

== system F16ASYM_Controlled_ACC/Primary Controller/P controller + adaptive Isolated NN/On-line (adaptive) multi-layer NNs SIMPL/Roll NN/Roll 2HL NN ==
  note: Be careful with dimensions of inputs!!!
      | NORMALIZATION!!!
  v_ad^ prev : Inport
  p_chanel vars : Inport  Port=2
  All_meas : Inport  Port=3
  Roll_learning rate : Inport  Port=4
  Roll reg param : Inport  Port=5
  " " : ToWorkspace  VariableName=Theta_3_roll_last  SampleTime=-1
      settings: MaxDataPoints=1
  "  " : Memory  X0=Theta_3_roll_last
  "   " : Memory  X0=Theta_2_roll_last
  B : Constant
  Bus Selector1 : BusSelector  OutputSignals=p_err,p_sf,p_sf_dot,K_b_p
  Bus Selector2 : BusSelector  OutputSignals=signal1.Alt meas (m),signal2.Mach,signal1.AoA meas (rad),signal1.SS meas (rad),signal1.omega_b meas (rad/s)
  Constant : Constant
  Constant2 : Constant
  Display : Display
  Divide : Product  Inputs=**
  Divide1 : Product  Inputs=**
  Divide2 : Product  Inputs=*/
  Gain : Gain  Gain=1/15000
  Memory2 : Memory  X0=Theta_1_roll_last
  Mux : Mux  Inputs=12
  Roll Multilayer NN : MATLAB Function  TreatAsAtomicUnit=on
  Scope : Scope
      settings: YMin=-14  YMax=4  SaveName=ScopeData16
  Selector : Selector  InputPortWidth=3  IndexOptions=Index vector (dialog)  Indices=3  OutputSizes=1
  Terminator : Terminator
  Terminator1 : Terminator
  To Workspace : ToWorkspace  VariableName=Theta_1_roll_last  SampleTime=-1
      settings: MaxDataPoints=1
  To Workspace1 : ToWorkspace  VariableName=Theta_2_roll_last  SampleTime=-1
      settings: MaxDataPoints=1
  v_ad_comp : Outport
  wires:
  Roll Multilayer NN/3(Z_norm_unit) -> Terminator1/1
  Mux/1 -> Roll Multilayer NN/1(X_bar), Scope/1, Display/1
  Roll reg param/1 -> Roll Multilayer NN/6(Roll_reg_param)
  Roll_learning rate/1 -> Roll Multilayer NN/5(Roll_learnign_rate)
  Memory2/1 -> Roll Multilayer NN/7(Theta_1)
  Roll Multilayer NN/5(Theta_2_update) -> "   "/1, To Workspace1/1
  "  "/1 -> Roll Multilayer NN/9(Theta_3)
  Roll Multilayer NN/6(Theta_3_update) -> " "/1, "  "/1
  Bus Selector2/2 -> Mux/3, Divide/1, Divide/2  "<Mach>"
  Constant2/1 -> Divide2/1
  Bus Selector1/4 -> Divide2/2  "<K_b_p>"
  Divide2/1 -> [P]
  Roll Multilayer NN/2(v_ad) -> Terminator/1
  Roll Multilayer NN/4(Theta_1_update) -> Memory2/1, To Workspace/1
  v_ad^ prev/1 -> Mux/12
  [P] -> Roll Multilayer NN/3(P)
  B/1 -> Roll Multilayer NN/4(B)
  "   "/1 -> Roll Multilayer NN/8(Theta_2)
  Roll Multilayer NN/1(v_ad_comp) -> v_ad_comp/1
  Selector/1 -> Mux/8
  Bus Selector2/5 -> Selector/1  "<omega_b meas (rad/s)>"
  Gain/1 -> Mux/2
  Bus Selector2/4 -> Mux/7  "<SS meas (rad)>"
  Divide1/1 -> Mux/6
  Bus Selector2/3 -> Mux/5, Divide1/1, Divide1/2  "<AoA meas (rad)>"
  Divide/1 -> Mux/4
  Bus Selector2/1 -> Gain/1  "<Alt meas (m)>"
  All_meas/1 -> Bus Selector2/1
  Constant/1 -> Mux/1
  Bus Selector1/1 -> Roll Multilayer NN/2(e), Mux/9  "<p_err>"
  Bus Selector1/3 -> Mux/11  "<p_sf_dot>"
  Bus Selector1/2 -> Mux/10  "<p_sf>"
  p_chanel vars/1 -> Bus Selector1/1

== system F16ASYM_Controlled_ACC/Primary Controller/P controller + adaptive Isolated NN/On-line (adaptive) multi-layer NNs SIMPL/Yaw Chanel/Yaw HL NN ==
  note: Be careful with dimensions of inputs!!!
      | NORMALIZATION!!!
  v_ad^ prev : Inport
  Yaw_chanel vars : Inport  Port=2
  All_meas : Inport  Port=3
  Yaw_learning rate : Inport  Port=4
  Yaw reg param : Inport  Port=5
  Bus Selector1 : BusSelector  OutputSignals=beta_chanel vars.beta_err,r_chanel vars.r_err,beta_chanel vars.beta_sf,beta_chanel vars.beta_sf_dot,r_chanel vars.r_sf_dot,beta_chanel vars.K_b_beta,r_chanel vars.K_b_r
  Bus Selector2 : BusSelector  OutputSignals=signal1.Alt meas (m),signal2.Mach,signal1.AoA meas (rad),signal1.Euler meas (rad)
  Constant : Constant
  Constant1 : Constant  Value=[0;1]
  Display : Display
  Divide : Product  Inputs=**
  Gain : Gain  Gain=1/15000
  Memory2 : Memory  X0=V_yaw_last
  Memory3 : Memory  X0=W_yaw_last
  Mux : Mux  Inputs=12
  Mux1 : Mux  Inputs=2
  Mux2 : Mux  Inputs=2
  Scope : Scope
      settings: YMin=-0.25  YMax=3.75  SaveName=ScopeData17
  Selector : Selector  InputPortWidth=3  IndexOptions=Index vector (dialog)  Indices=1  OutputSizes=1
  Terminator : Terminator
  Terminator1 : Terminator
  To Workspace : ToWorkspace  VariableName=V_yaw_last  SampleTime=-1
      settings: MaxDataPoints=1
  To Workspace1 : ToWorkspace  VariableName=W_yaw_last  SampleTime=-1
      settings: MaxDataPoints=1
  Yaw NN : MATLAB Function  TreatAsAtomicUnit=on
  v_ad_comp : Outport
  wires:
  Yaw NN/3(Z_norm_unit) -> Terminator1/1
  Mux/1 -> Yaw NN/1(X_bar), Scope/1, Display/1
  Bus Selector1/3 -> Mux/9  "<beta_sf>"
  Bus Selector1/1 -> Mux/7, Mux1/1  "<beta_err>"
  Bus Selector1/4 -> Mux/10  "<beta_sf_dot>"
  Bus Selector1/2 -> Mux/8, Mux1/2  "<r_err>"
  Bus Selector1/5 -> Mux/11  "<r_sf_dot>"
  Selector/1 -> Mux/6
  Bus Selector2/3 -> Mux/5  "<AoA meas (rad)>"
  Bus Selector2/2 -> Mux/3, Divide/1, Divide/2  "<Mach>"
  Gain/1 -> Mux/2
  Bus Selector2/4 -> Selector/1  "<Euler meas (rad)>"
  Yaw NN/2(v_ad) -> Terminator/1
  Yaw NN/5(V_update) -> To Workspace/1, Memory2/1
  v_ad^ prev/1 -> Mux/12
  [Ks] -> Yaw NN/3(Ks)
  Constant1/1 -> Yaw NN/4(B)
  Memory3/1 -> Yaw NN/7(W)
  Memory2/1 -> Yaw NN/8(V)
  Yaw NN/4(W_update) -> To Workspace1/1, Memory3/1
  Yaw NN/1(v_ad_comp) -> v_ad_comp/1
  Yaw_chanel vars/1 -> Bus Selector1/1
  Yaw_learning rate/1 -> Yaw NN/5(Long_learnign_rate)
  Yaw reg param/1 -> Yaw NN/6(Long_reg_param)
  Constant/1 -> Mux/1
  All_meas/1 -> Bus Selector2/1
  Bus Selector2/1 -> Gain/1  "<Alt meas (m)>"
  Divide/1 -> Mux/4
  Mux1/1 -> Yaw NN/2(e)  "e"
  Bus Selector1/7 -> Mux2/2  "<K_b_r>"
  Bus Selector1/6 -> Mux2/1  "<K_b_beta>"
  Mux2/1 -> [Ks]

== system F16ASYM_Controlled_ACC/Primary Controller/PI Primary Controller/Longitudinal Controller: AoA or A_w_z/Longitudinal controller in A_w_z/Accel rate --> AoA rate! ==
  A_w_z dot : Inport
  All_meas : Inport  Port=2
  1/a_1 : Gain  Gain=1/a1
  Bus Selector : BusSelector  OutputSignals=signal2.q (Pa)
  Divide : Product  Inputs=**
  Divide1 : Product  Inputs=**
  Divide2 : Product  Inputs=*/
  S : Constant  Value=27.87
  mass : Constant  Value=9295.44
  alpha_dot des : Outport
  wires:
  1/a_1/1 -> alpha_dot des/1  "ALPHA_DOT"
  All_meas/1 -> Bus Selector/1
  Divide2/1 -> 1/a_1/1
  Divide/1 -> Divide2/2
  Divide1/1 -> Divide2/1
  mass/1 -> Divide1/2
  Bus Selector/1 -> Divide/2  "<q (Pa)>"
  S/1 -> Divide/1
  A_w_z dot/1 -> Divide1/1

== matlab function F16ASYM_Controlled_ACC/Primary Controller/P controller + adaptive Isolated NN/On-line (adaptive) multi-layer NNs/Roll NN/Roll 2HL NN/Roll Multilayer NN ==
  data: X_bar input size=[12,1]; v_ad_comp output; e input size=1; P input; B input; Roll_learnign_rate input size=1; Roll_reg_param input size=1; Theta_1 input size=[30,12]; Theta_2 input size=[20,31]; Theta_3 input size=[1,21]; v_ad output; Z_norm_unit output; T_sim parameter; Theta_1_update output; Theta_2_update output; Theta_3_update output
function [v_ad_comp,v_ad,Z_norm_unit,Theta_1_update,Theta_2_update,Theta_3_update]  = Roll_ML_NN(X_bar,e,P,B,Roll_learnign_rate, Roll_reg_param,Theta_1,Theta_2,Theta_3,T_sim)

%% Compute prelimiary parameters
zeta= e'*P*B;

%% Feedforward. Layers: Sigmoidal, linear, linear

a2=[1 ;  sigmoid( Theta_1*X_bar )]; % Sigmoidal
a3=[1 ;  (Theta_2*a2)]; % Linear
% z4=Theta_3*a3;
% a4 = z4; % Linear
% v_ad =a4;

% Backward
% % delta4=zeta; % In this particular case of adaptive NN, this error is a weighted tracking error
delta3=Theta_3'*zeta;
delta2=Theta_2'*delta3(2:end).*(a2.*(ones(size(a2))-a2)); 


%% Compute the gradients or adaptation laws
Gamma_Theta_3= Roll_learnign_rate; %  learnign rate
Gamma_Theta_2 = Roll_learnign_rate; % learning rate
Gamma_Theta_1= Roll_learnign_rate; % learning rate
lambda = Roll_reg_param;    % Regularization constant

% % Theta_1_dot=zeros(size(Theta_1));
% % Theta_2_dot=zeros(size(Theta_2));
% % Theta_3_dot=zeros(size(Theta_3));

Theta_3_dot = -Gamma_Theta_3*zeta*a3' ;
Theta_3_dot(:,2:end) =  Theta_3_dot(:,2:end) - Gamma_Theta_3*lambda*norm(zeta).*Theta_3(:,2:end);

Theta_2_dot= -Gamma_Theta_2*( delta3(2:end)*a2'   + lambda*norm(zeta).*Theta_2);
Theta_2_dot(:,2:end) =  Theta_2_dot(:,2:end) - Gamma_Theta_2*lambda*norm(zeta).*Theta_2(:,2:end);

Theta_1_dot= -Gamma_Theta_1*( delta2(2:end)*X_bar'   + lambda*norm(zeta).*Theta_1);
Theta_1_dot(:,2:end) =  Theta_1_dot(:,2:end) - Gamma_Theta_1*lambda*norm(zeta).*Theta_1(:,2:end);


%% Adaptation
Theta_1_update = Theta_1 + T_sim*Theta_1_dot;
Theta_2_update = Theta_2 + T_sim*Theta_2_dot;
Theta_3_update = Theta_3 + T_sim*Theta_3_dot;

%% re-compute v_ad

a2=[1 ;  sigmoid( Theta_1_update*X_bar )]; % Sigmoidal
a3=[1 ;  (Theta_2_update*a2)]; % Linear
v_ad=Theta_3_update*a3;


%% Compute v_ad_comp
% Z = blkdiag( Theta_1_update , Theta_2_update , Theta_3_update );

Z =  [ Theta_1_update, zeros(size(Theta_1_update,1),size(Theta_2_update,2)) , zeros(size(Theta_1_update,1),size(Theta_3_update,2));
            zeros(size(Theta_2_update,1),size(Theta_1_update,2)) , Theta_2_update , zeros(size(Theta_2_update,1),size(Theta_3_update,2)) ;
            zeros(size(Theta_3_update,1),size(Theta_1_update,2)),zeros(size(Theta_3_update,1),size(Theta_2_update,2)),  Theta_3_update ];

Z_norm = norm(Z,'fro');
Z_max = min(size(Theta_1))*min(size(Theta_2))*min(size(Theta_3));
Z_norm_unit = Z_norm;

K_r0= 0.02;
K_r1= 0;
v_r0 = -K_r0*zeta;
v_r1 = -K_r1*(Z_norm+Z_max)*zeta;

v_ad_comp = v_ad + v_r1 +v_r0;


end

== matlab function F16ASYM_Controlled_ACC/Faults injection/MATLAB Function ==
  data: reconfig_params output; Delta_mass input; Delta_S_L input; Delta_S_R input; Delta_S_Fin input; xcg input; Delta_J input; Eff input; Deltas_coef input
function reconfig_params  = Reconfig_params(Delta_mass,Delta_S_L,Delta_S_R,Delta_S_Fin,xcg,Delta_J,Eff,Deltas_coef)

reconfig_params= zeros(19,1);

S_L  = 27.87/2;
S_R = 27.87/2;
S_fin = 6.578;

if size(Eff,2)==7
    Eff=Eff';
end
if size(Deltas_coef,2)==3
    Deltas_coef=Deltas_coef';
end

reconfig_params(1)= 9295.44*(1+Delta_mass); % mass
reconfig_params(2) = S_L*0.3 + 0.7*S_L*(1-Delta_S_L); % S_current_L. Split between 0.2 and 0.8 because it would imposible to lose a 100% which is part of fuselage 
reconfig_params(3) = S_R*0.3 + 0.7*S_R*(1-Delta_S_R); % S_current_R
reconfig_params(4) = S_fin*0.1 + 0.9*S_fin*(1-Delta_S_Fin);   % S_fin_current
reconfig_params(5) = xcg;  % xcg
reconfig_params(6) = 75673.6*(1+Delta_J(1)); % Jy
reconfig_params(7) = 1331.4*(1+Delta_J(2));  % Jxz
reconfig_params(8)  = 85552.1*(1+Delta_J(3)); % Jz
reconfig_params(9) = 12874.8*(1+Delta_J(4));   % Jx
reconfig_params(10:16)  = Eff; % Effectiveness
reconfig_params(17:19)  = Deltas_coef; %Deltas lift, drag and pitching moment

end

== matlab function F16ASYM_Controlled_ACC/Primary Controller/P controller + adaptive Isolated NN/On-line (adaptive) multi-layer NNs/Roll NN/Roll 1HL NN/Roll NN ==
  data: X_bar input size=[12,1]; v_ad_comp output; e input; P input; B input; Roll_learnign_rate input size=1; Roll_reg_param input size=1; W input size=[1,31]; V input size=[30,12]; v_ad output; Z_norm_unit output; T_sim parameter; W_update output size=[1,31]; V_update output size=[30,12]
function [v_ad_comp,v_ad,Z_norm_unit,W_update,V_update]  = Roll_NN(X_bar,e,P,B,Roll_learnign_rate,Roll_reg_param,W,V,T_sim)

%% Compute prelimiary parametes
zeta= e'*P*B;
s=zeros(30,1);
z=s;
%% Feedforward
z = V*X_bar;
s=sigmoid(V*X_bar);

sigma = [1 ; s ];
% v_ad = W*sigma;

sigma_grad = (sigma.*(ones(size(sigma))-sigma));

%% Compute the gradients or adaptation laws
Gamma_w= Roll_learnign_rate; % W learnign rate
Gamma_v= Roll_learnign_rate; %V learning rate
lambda = Roll_reg_param;

V_dot=zeros(size(V));
W_dot=zeros(size(W'));

W_dot= -Gamma_w*(  (sigma - sigma_grad.*[1;z] ).*zeta  );
W_dot(2:end,1)= W_dot(2:end,1) - Gamma_w*lambda*norm(zeta)*(W(:,2:end))';

M = W'*zeta.*sigma_grad ;
V_dot= -Gamma_v*( M(2:end)*X_bar'  );
V_dot(:,2:end)= V_dot(:,2:end) - Gamma_v*lambda*norm(zeta).*V(:,2:end);


% Other way: Based on notes of Andrew NG
% % % W_dot=zeros(size(W));
% % % delta2=W'*zeta.*sigma_grad;
% % % 
% % % V_dot = - Gamma_v*( delta2(2:end)*X_bar');
% % % V_dot(:,2:end)= V_dot(:,2:end) - Gamma_v*lambda*norm(zeta).*V(:,2:end);
% % % 
% % % W_dot = - Gamma_w*( zeta*sigma');
% % % W_dot(:,2:end)= W_dot(:,2:end) - Gamma_w*lambda*norm(zeta)*(W(:,2:end));
% % % 
% % % W_dot = W_dot';


%% Adaptation
W_update = W + T_sim*W_dot';
V_update = V + T_sim*V_dot;

%% re-compute v_ad

z = V*X_bar;
s=sigmoid(V*X_bar);

sigma = [1 ; s(:,1) ];
v_ad = W*sigma;

%% Compute v_ad_comp
Z = [ V,zeros(size(V,1),size(W,2));
    zeros(size(W,1),size(V,2)),W];
    
Z_norm = norm(Z,'fro');
Z_max = 2*min(size(W,1),size(W,2) )*min( size(V,1),size(V,2) );
Z_norm_unit = Z_norm;

K_r0= 0;
K_r1= 0;
v_r0 = -K_r0*zeta;
v_r1 = -K_r1*(Z_norm+Z_max)*zeta;
v_ad_comp = v_ad + v_r1 +v_r0;

% % K_r1= 1;
% % v_r1 = - K_r1*(Z_norm+Z_max)*zeta;
% % 
% % v_ad_comp = v_ad + v_r1 ;



end

== matlab function F16ASYM_Controlled_ACC/Primary Controller/P controller + adaptive Isolated NN/On-line (adaptive) multi-layer NNs/Long Chanel/Long HL NN AoA/Long NN ==
  data: X_bar input size=[10,1]; v_ad_comp output; e input; Ks input; B input; Long_learnign_rate input size=1; Long_reg_param input size=1; W input size=[1,31]; V input size=[30,10]; v_ad output; Z_norm_unit output; T_sim parameter; W_update output; V_update output
function [v_ad_comp,v_ad,Z_norm_unit,W_update,V_update]  = Long_AoA_NN(X_bar,e, Ks,B,Long_learnign_rate,Long_reg_param,W,V,T_sim)

%% Compute prelimiary parametes Ks(1)=K_b_alpha  and Ks(2) = K_b_q
P = [   1/Ks(1) , 1/(Ks(1)^2+Ks(1)*Ks(2));
     1/(Ks(1)^2+Ks(1)*Ks(2)) ,(Ks(1)^2+Ks(1)*Ks(2)+1)/(Ks(2)^2*Ks(1)+Ks(2)*Ks(1)^2) ];
zeta= e'*P*B;
s=zeros(30,1);
z=s;
%% Feedforward
z = V*X_bar;
s=sigmoid(V*X_bar);

sigma = [1 ; s ];
% v_ad = W*sigma;

sigma_grad = (sigma.*(ones(size(sigma))-sigma));

%% Compute the gradients or adaptation laws
Gamma_w= Long_learnign_rate; % W learnign rate
Gamma_v= Long_learnign_rate; %V learning rate
lambda = Long_reg_param;

V_dot=zeros(size(V));
W_dot=zeros(size(W'));

W_dot= -Gamma_w*(  (sigma - sigma_grad.*[1;z] ).*zeta  );
W_dot(2:end,1)= W_dot(2:end,1) - Gamma_w*lambda*norm(zeta)*(W(:,2:end))';

M = W'*zeta.*sigma_grad ;
V_dot= -Gamma_v*( M(2:end)*X_bar'  );
V_dot(:,2:end)= V_dot(:,2:end) - Gamma_v*lambda*norm(zeta).*V(:,2:end);


% % % Other way: Based on notes of Andrew NG
% % W_dot=zeros(size(W));
% % delta2=W'*zeta.*sigma_grad;
% % 
% % V_dot = - Gamma_v*( delta2(2:end)*X_bar');
% % V_dot(:,2:end)= V_dot(:,2:end) - Gamma_v*lambda*norm(zeta).*V(:,2:end);
% % 
% % W_dot = - Gamma_w*( zeta*sigma');
% % W_dot(:,2:end)= W_dot(:,2:end) - Gamma_w*lambda*norm(zeta)*(W(:,2:end));
% % 
% % W_dot = W_dot';


%% Adaptation
W_update = W + T_sim*W_dot';
V_update = V + T_sim*V_dot;

%% re-compute v_ad

z = V*X_bar;
s=sigmoid(V*X_bar);

sigma = [1 ; s(:,1) ];
v_ad = W*sigma;

%% Compute v_ad_comp
Z = [ V,zeros(size(V,1),size(W,2));
    zeros(size(W,1),size(V,2)),W];
    
Z_norm = norm(Z,'fro');
Z_max = 2*min(size(W,1),size(W,2) )*min( size(V,1),size(V,2) );
Z_norm_unit = Z_norm;

K_r0= 0.02;
K_r1= 0;
v_r0 = -K_r0*zeta;
v_r1 = -K_r1*(Z_norm+Z_max)*zeta;

v_ad_comp = v_ad + v_r1 +v_r0;


end

== matlab function F16ASYM_Controlled_ACC/Primary Controller/P controller + adaptive Isolated NN/On-line (adaptive) multi-layer NNs/Long Chanel/Long HL NN A_w_z/Long NN ==
  data: X_bar input size=[10,1]; v_ad_comp output; e input; F input; Ks input; B input; Long_learnign_rate input size=1; Long_reg_param input size=1; W input size=[1,31]; V input size=[30,10]; v_ad output; Z_norm_unit output; T_sim parameter; W_update output; V_update output
function [v_ad_comp,v_ad,Z_norm_unit,W_update,V_update]  = Long_AoA_NN(X_bar,e, F, Ks,B,Long_learnign_rate,Long_reg_param,W,V,T_sim)

%% Compute prelimiary parametes Ks(1)=K_b_alpha  and Ks(2) = K_b_q
P = [   1/Ks(1) , F/(Ks(1)^2+Ks(1)*Ks(2));
     1/(Ks(1)^2+Ks(1)*Ks(2)) ,(Ks(1)^2+Ks(1)*Ks(2)+F^2)/(Ks(2)^2*Ks(1)+Ks(2)*Ks(1)^2) ];
zeta= e'*P*B;
s=zeros(30,1);
z=s;
%% Feedforward
z = V*X_bar;
s=sigmoid(V*X_bar);

sigma = [1 ; s ];
% v_ad = W*sigma;

sigma_grad = (sigma.*(ones(size(sigma))-sigma));

%% Compute the gradients or adaptation laws
Gamma_w= Long_learnign_rate; % W learnign rate
Gamma_v= Long_learnign_rate; %V learning rate
lambda = Long_reg_param;

V_dot=zeros(size(V));
W_dot=zeros(size(W'));

W_dot= -Gamma_w*(  (sigma - sigma_grad.*[1;z] ).*zeta  );
W_dot(2:end,1)= W_dot(2:end,1) - Gamma_w*lambda*norm(zeta)*(W(:,2:end))';

M = W'*zeta.*sigma_grad ;
V_dot= -Gamma_v*( M(2:end)*X_bar'  );
V_dot(:,2:end)= V_dot(:,2:end) - Gamma_v*lambda*norm(zeta).*V(:,2:end);


% % % Other way: Based on notes of Andrew NG
% % W_dot=zeros(size(W));
% % delta2=W'*zeta.*sigma_grad;
% % 
% % V_dot = - Gamma_v*( delta2(2:end)*X_bar');
% % V_dot(:,2:end)= V_dot(:,2:end) - Gamma_v*lambda*norm(zeta).*V(:,2:end);
% % 
% % W_dot = - Gamma_w*( zeta*sigma');
% % W_dot(:,2:end)= W_dot(:,2:end) - Gamma_w*lambda*norm(zeta)*(W(:,2:end));
% % 
% % W_dot = W_dot';


%% Adaptation
W_update = W + T_sim*W_dot';
V_update = V + T_sim*V_dot;

%% re-compute v_ad

z = V*X_bar;
s=sigmoid(V*X_bar);

sigma = [1 ; s(:,1) ];
v_ad = W*sigma;

%% Compute v_ad_comp
Z = [ V,zeros(size(V,1),size(W,2));
    zeros(size(W,1),size(V,2)),W];
    
Z_norm = norm(Z,'fro');
Z_max = 2*min(size(W,1),size(W,2) )*min( size(V,1),size(V,2) );
Z_norm_unit = Z_norm/Z_max;

K_r0= 0.1;
K_r1= 0.001;
v_r0 = -K_r0*zeta;
v_r1 = -K_r1*(Z_norm+Z_max)*zeta;

v_ad_comp = v_ad + v_r1 +v_r0;


end

== matlab function F16ASYM_Controlled_ACC/Primary Controller/P controller + adaptive Isolated NN/Sigmoid /MATLAB Function ==
  data: u input; y output; a input
function y = sigmoid_a(u,a)

y = 2.0 ./ (1.0 + exp(-a*u(1:3)))-1;
